simulink model "SwarmSystem_2021b"  (R2021b)
settings: Solver=VariableStepAuto  StartTime=0.0  StopTime=10.0  RelTol=1e-3
values from neighbouring files (symbols this model uses):
  dt = 0.01    [init_params.m]
  initial_state_x0 = Simulink.Parameter(initial_state_x0)    [init_params.m]    (also in single_model_verification_script.m = [W0; R0; dP0; P0]; team_model_conf_comp_script.m = [W0; R0; dP0; P0]; team_model_tethered_tilt.m = [W0; R0; dP0; P0]; team_model_tracking_script.m = [W0; R0; dP0; P0])
undefined symbols (not defined in the file or in its folder): ctrl_params, drone_params, env_params, initial_state_z0
libraries: dspindex x15
settings Model: Creator=NTU  LastModifiedBy=NTU
settings DataIOCC: SaveFinalState=on  SaveState=on
settings DebuggingCC: UnconnectedInputMsg=none  UnconnectedOutputMsg=none  UnconnectedLineMsg=none
settings ModelReferenceCC: EnableRefExpFcnMdlSchedulingChecks=off
settings RTWCC: DLArmComputeVersion=20.02.1

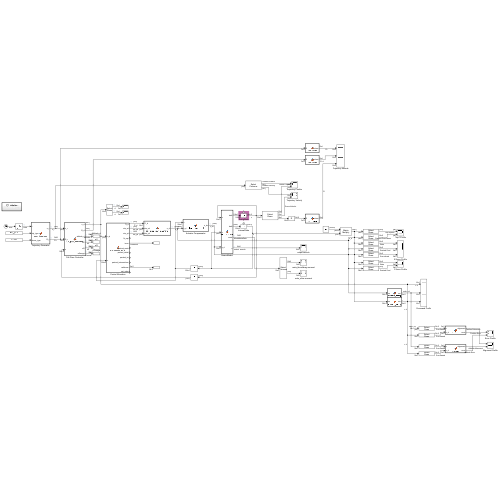
[thumbnail: Simulink's stored preview of the top-level diagram]
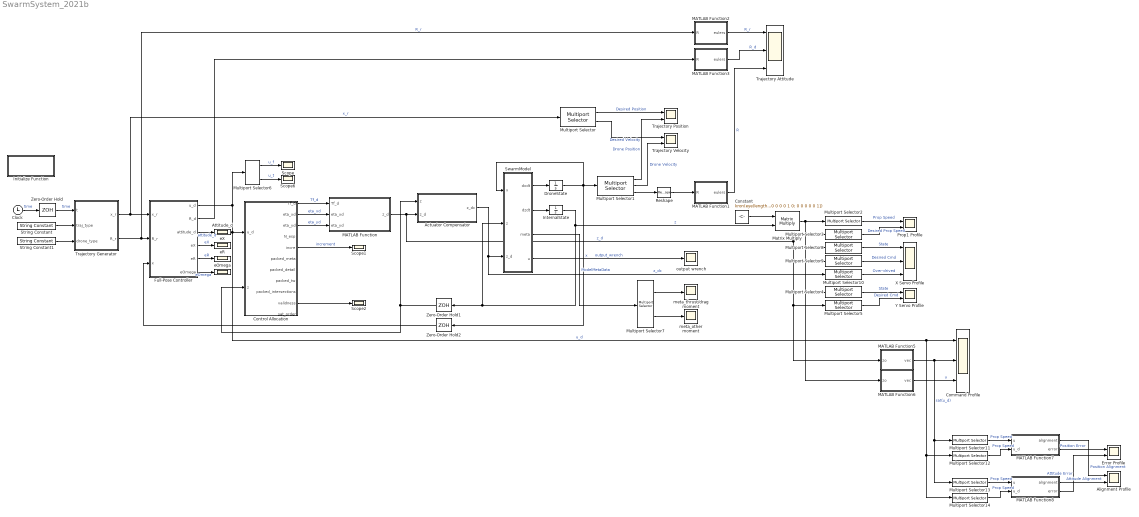
== system SwarmSystem_2021b ==
  Actuator Compensator : MATLAB Function  TreatAsAtomicUnit=on
  Alignment Profile : Scope  NumInputPorts=2
  Attitude_d : Scope
  Clock : Clock
  Command Profile : Scope  NumInputPorts=3
  Constant : Constant  Value=kron(eye(length(drone_params.psi)), [1 0 0 0 0 0;0 0 1 0 0 0; 0 0 0 0 1 0; 0 0 0 0 0 1])  VectorParams1D=off
  Control Allocation : MATLAB Function  TreatAsAtomicUnit=on
  DroneState : Integrator  InitialCondition=zeros([18 1])  ContinuousStateAttributes='x'
  Error Profile : Scope  NumInputPorts=2
  Full-Pose Controller : MATLAB Function  TreatAsAtomicUnit=on
  Initialize Function : Subsystem  TreatAsAtomicUnit=on
  InternalState : Integrator  InitialCondition=zeros([6*length(drone_params.psi) 1])  ContinuousStateAttributes='z'
  MATLAB Function : MATLAB Function  TreatAsAtomicUnit=on
  MATLAB Function1 : MATLAB Function  TreatAsAtomicUnit=on
  MATLAB Function2 : MATLAB Function  TreatAsAtomicUnit=on
  MATLAB Function3 : MATLAB Function  TreatAsAtomicUnit=on
  MATLAB Function5 : MATLAB Function  TreatAsAtomicUnit=on
  MATLAB Function6 : MATLAB Function  TreatAsAtomicUnit=on
  MATLAB Function7 : MATLAB Function  TreatAsAtomicUnit=on
  MATLAB Function8 : MATLAB Function  TreatAsAtomicUnit=on
  Matrix Multiply : Product  Multiplication=Matrix(*)
  Multiport Selector : dspindex/Multiport Selector  rowsOrCols=Columns  idxCellArray={ 1, 2 }  idxErrMode=Clip Index
  Multiport Selector1 : dspindex/Multiport Selector  rowsOrCols=Rows  idxCellArray={ [16:18], [13:15], [4:12] }  idxErrMode=Clip Index
  Multiport Selector10 : dspindex/Multiport Selector  rowsOrCols=Rows  idxCellArray={ [4 8 12 16 20 24 28 32 36]-3 }  idxErrMode=Clip Index
  Multiport Selector11 : dspindex/Multiport Selector  rowsOrCols=Rows  idxCellArray={ [1:3]}  idxErrMode=Clip Index
  Multiport Selector12 : dspindex/Multiport Selector  rowsOrCols=Rows  idxCellArray={ [1:3]}  idxErrMode=Clip Index
  Multiport Selector13 : dspindex/Multiport Selector  rowsOrCols=Rows  idxCellArray={ [4:6]}  idxErrMode=Clip Index
  Multiport Selector14 : dspindex/Multiport Selector  rowsOrCols=Rows  idxCellArray={ [4:6]}  idxErrMode=Clip Index
  Multiport Selector2 : dspindex/Multiport Selector  rowsOrCols=Rows  idxCellArray={ [4 8 12 16 20 24 28 32 36]-1 }  idxErrMode=Clip Index
  Multiport Selector3 : dspindex/Multiport Selector  rowsOrCols=Rows  idxCellArray={ [4 8 12 16 20 24 28 32 36]-1 }  idxErrMode=Clip Index
  Multiport Selector4 : dspindex/Multiport Selector  rowsOrCols=Rows  idxCellArray={ [4 8 12 16 20 24 28 32 36]-2 }  idxErrMode=Clip Index
  Multiport Selector5 : dspindex/Multiport Selector  rowsOrCols=Rows  idxCellArray={ [4 8 12 16 20 24 28 32 36]-2 }  idxErrMode=Clip Index
  Multiport Selector6 : dspindex/Multiport Selector  rowsOrCols=Rows  idxCellArray={ [1:3], [4:6] }  idxErrMode=Clip Index
  Multiport Selector7 : dspindex/Multiport Selector  rowsOrCols=Columns  idxCellArray={ [1:2], [3:5]}  idxErrMode=Clip Index
  Multiport Selector8 : dspindex/Multiport Selector  rowsOrCols=Rows  idxCellArray={ [4 8 12 16 20 24 28 32 36]-3 }  idxErrMode=Clip Index
  Multiport Selector9 : dspindex/Multiport Selector  rowsOrCols=Rows  idxCellArray={ [4 8 12 16 20 24 28 32 36]-3 }  idxErrMode=Clip Index
  Prop1 Profile : Scope  NumInputPorts=2
  Reshape : Reshape  OutputDimensionality=Customize  OutputDimensions=[3,3]
  Scope{,1..2,6} (4 alike) : Scope
  String Constant : StringConstant  String=traj_type
  String Constant1 : StringConstant  String="\"team\""
  SwarmModel : MATLAB Function  TreatAsAtomicUnit=on
  Trajectory Attitude : Scope  NumInputPorts=3
  Trajectory Generator : MATLAB Function  TreatAsAtomicUnit=on
  Trajectory Position : Scope  NumInputPorts=2
  Trajectory Velocity : Scope  NumInputPorts=2
  X Servo Profile : Scope  NumInputPorts=3
  Y Servo Profile : Scope  NumInputPorts=2
  Zero-Order Hold : ZeroOrderHold  SampleTime=dt
  Zero-Order Hold1 : ZeroOrderHold  SampleTime=dt
  Zero-Order Hold2 : ZeroOrderHold  SampleTime=dt
  eOmega : Scope
  eR : Scope
  eX : Scope
  meta_other moment : Scope
  meta_thrust/drag moment : Scope
  output wrench : Scope
  wires:
  SwarmModel/1(dxdt) -> DroneState/1
  Clock/1 -> Zero-Order Hold/1  "time"
  Trajectory Generator/1(x_r) -> Multiport Selector/1, Full-Pose Controller/1(x_r)  "x_r"
  Trajectory Generator/2(R_r) -> MATLAB Function2/1(R), Full-Pose Controller/2(R_r)  "R_r"
  Multiport Selector/1 -> Trajectory Position/1  "Desired Position"
  Multiport Selector1/1 -> Trajectory Position/2  "Drone Position"
  Multiport Selector1/2 -> Trajectory Velocity/2  "Drone Velocity"
  Multiport Selector/2 -> Trajectory Velocity/1  "Desired Velocity"
  Multiport Selector2/1 -> Prop1 Profile/1  "Prop Speed"
  SwarmModel/2(dzdt) -> InternalState/1
  Control Allocation/1(Tf_d) -> MATLAB Function/1(Tf_d)  "Tf_d"
  Control Allocation/2(eta_xd) -> MATLAB Function/2(eta_xd)  "eta_xd"
  Control Allocation/3(eta_yd) -> MATLAB Function/3(eta_yd)  "eta_yd"
  MATLAB Function/1(z_d) -> Multiport Selector3/1, MATLAB Function5/1(zo), Multiport Selector5/1, Multiport Selector9/1, Actuator Compensator/2(z_d)  "z_d"
  DroneState/1 -> SwarmModel/1(x), Zero-Order Hold2/1, Multiport Selector1/1  "x"
  InternalState/1 -> Zero-Order Hold1/1, SwarmModel/2(z), Matrix Multiply/2  "z"
  Multiport Selector6/1 -> Scope/1  "u_f"
  Multiport Selector6/2 -> Scope6/1  "u_t"
  MATLAB Function1/1(eulers) -> Trajectory Attitude/3  "R"
  Multiport Selector1/3 -> Reshape/1
  Reshape/1 -> MATLAB Function1/1(R)
  MATLAB Function2/1(eulers) -> Trajectory Attitude/1  "R_r"
  Full-Pose Controller/2(R_d) -> MATLAB Function3/1(R)
  MATLAB Function3/1(eulers) -> Trajectory Attitude/2  "R_d"
  Constant/1 -> Matrix Multiply/1
  MATLAB Function6/1(vec) -> Command Profile/3  "u"
  Multiport Selector3/1 -> Prop1 Profile/2  "Desired Prop Speed"
  Multiport Selector8/1 -> X Servo Profile/1  "State"
  Multiport Selector9/1 -> X Servo Profile/2  "Desired Cmd"
  Multiport Selector5/1 -> Y Servo Profile/2  "Desired Cmd"
  Multiport Selector4/1 -> Y Servo Profile/1  "State"
  Matrix Multiply/1 -> MATLAB Function6/1(zo), Multiport Selector4/1, Multiport Selector8/1, Multiport Selector2/1
  Zero-Order Hold/1 -> Trajectory Generator/1(t)  "time"
  Actuator Compensator/1(z_dc) -> Multiport Selector10/1, SwarmModel/3(z_d)  "z_dc"
  Multiport Selector10/1 -> X Servo Profile/3  "Over-drived"
  Zero-Order Hold1/1 -> Actuator Compensator/1(z), Control Allocation/2(z)
  Zero-Order Hold2/1 -> Full-Pose Controller/3(x)
  Multiport Selector11/1 -> MATLAB Function7/1(u)  "Prop Speed"
  Multiport Selector12/1 -> MATLAB Function7/2(u_d)  "Prop Speed"
  Multiport Selector14/1 -> MATLAB Function8/2(u_d)  "Prop Speed"
  Multiport Selector13/1 -> MATLAB Function8/1(u)  "Prop Speed"
  Full-Pose Controller/1(u_d) -> Multiport Selector12/1, Multiport Selector14/1, Command Profile/1, Control Allocation/1(u_d), Multiport Selector6/1  "u_d"
  MATLAB Function5/1(vec) -> Multiport Selector13/1, Multiport Selector11/1, Command Profile/2  "sat(u_d)"
  MATLAB Function7/2(error) -> Error Profile/1  "Position Error"
  MATLAB Function8/2(error) -> Error Profile/2  "Attitude Error"
  MATLAB Function7/1(alignment) -> Alignment Profile/1  "Position Alignment"
  MATLAB Function8/1(alignment) -> Alignment Profile/2  "Attitude Alignment"
  Control Allocation/5(incre) -> Scope1/1  "increment"
  Control Allocation/10(validness) -> Scope2/1
  String Constant/1 -> Trajectory Generator/2(traj_type)
  String Constant1/1 -> Trajectory Generator/3(drone_type)
  Full-Pose Controller/4(eX) -> eX/1  "eX"
  Full-Pose Controller/6(eOmega) -> eOmega/1  "eOmega"
  Full-Pose Controller/5(eR) -> eR/1  "eR"
  Full-Pose Controller/3(attitude_d) -> Attitude_d/1  "attitude_d"
  Multiport Selector7/2 -> meta_other moment/1
  Multiport Selector7/1 -> meta_thrust/drag moment/1
  SwarmModel/3(meta) -> Multiport Selector7/1  "ModelMetaData"
  SwarmModel/4(u) -> output wrench/1  "output_wrench"

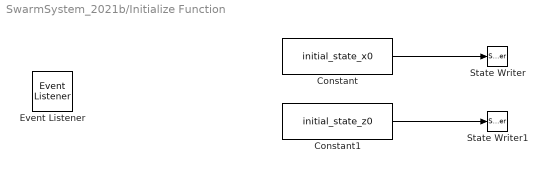
== system SwarmSystem_2021b/Initialize Function ==
  Constant : Constant  Value=initial_state_x0  VectorParams1D=off
  Constant1 : Constant  Value=initial_state_z0  VectorParams1D=off
  Event Listener : EventListener  DisableCoverage=on  EventName=reset
  State Writer : StateWriter  StateOwnerBlock=../../DroneState  StateName=x
  State Writer1 : StateWriter  StateOwnerBlock=../../InternalState  StateName=z
  wires:
  Constant/1 -> State Writer/1
  Constant1/1 -> State Writer1/1

== matlab function SwarmSystem_2021b/MATLAB Function2 ==
  data: R input; eulers output
function eulers = rotm2euler(R)
    psi = atan2(-R(1, 2), R(2, 2));    
    phi = atan2(R(3, 2), sqrt(abs(1-R(3, 2).^2)));
    theta = atan2(-R(3, 1), R(3, 3));
    eulers = [psi phi theta]';
end

== matlab function SwarmSystem_2021b/MATLAB Function3 ==
  data: R input; eulers output
function eulers = rotm2euler(R)
    psi = atan2(-R(1, 2), R(2, 2));    
    phi = atan2(R(3, 2), sqrt(abs(1-R(3, 2).^2)));
    theta = atan2(-R(3, 1), R(3, 3));
    eulers = [psi phi theta]';
end

== matlab function SwarmSystem_2021b/MATLAB Function5 ==
  data: zo input; drone_params parameter; vec output; env_params parameter
function vec = actuator_mixing(zo, drone_params, env_params)
    %% Parameters
    g = env_params.g; % gravity
    rho = env_params.rho; % kg/m3
    prop_d = env_params.prop_d; % 8 inch = 20.3 cm
    
    CT_u = env_params.CT_u; % upper propeller thrust coefficient
    CT_l = env_params.CT_l; % lower propeller thrust coefficient
    CP_u = env_params.CP_u; % upper propeller drag coefficient
    CP_l = env_params.CP_l; % lower propeller drag coefficient

    pos = drone_params.pos;
    psi = drone_params.psi;
    n = length(psi);

    Tf = zeros([n 1]);
    eta_x = zeros([n 1]);
    eta_y = zeros([n 1]);

    beta_allo = [CT_u CT_l; prop_d * CP_u -prop_d * CP_l];
    P_prop = rho * prop_d^4 * beta_allo;

    for i = 1:n
        % Actuator Model
        zi = zo(4 * (i - 1) + 1 : 4 * i);
        TfTdi = P_prop * zi(3:4, 1).^2;
        Tf(i) = TfTdi(1);
        eta_x(i) = zi(1);
        eta_y(i) = zi(2);
    end

    M = get_M(n, psi, pos);
    fi = get_f(eta_x, eta_y, Tf);
    vec = M * fi;
end

== matlab function SwarmSystem_2021b/MATLAB Function6 ==
  data: zo input; drone_params parameter; vec output; env_params parameter
function vec = actuator_mixing(zo, drone_params, env_params)
    %% Parameters
    g = env_params.g; % gravity
    rho = env_params.rho; % kg/m3
    prop_d = env_params.prop_d; % 8 inch = 20.3 cm
    
    CT_u = env_params.CT_u; % upper propeller thrust coefficient
    CT_l = env_params.CT_l; % lower propeller thrust coefficient
    CP_u = env_params.CP_u; % upper propeller drag coefficient
    CP_l = env_params.CP_l; % lower propeller drag coefficient

    pos = drone_params.pos;
    psi = drone_params.psi;
    n = length(psi);

    Tf = zeros([n 1]);
    eta_x = zeros([n 1]);
    eta_y = zeros([n 1]);

    beta_allo = [CT_u CT_l; prop_d * CP_u -prop_d * CP_l];
    P_prop = rho * prop_d^4 * beta_allo;

    for i = 1:n
        % Actuator Model
        zi = zo(4 * (i - 1) + 1 : 4 * i);
        TfTdi = P_prop * zi(3:4, 1).^2;
        Tf(i) = TfTdi(1);
        eta_x(i) = zi(1);
        eta_y(i) = zi(2);
    end

    M = get_M(n, psi, pos);
    fi = get_f(eta_x, eta_y, Tf);
    vec = M * fi;
end

== matlab function SwarmSystem_2021b/Actuator Compensator ==
  settings: updateMethod=DISCRETE  sampleTime=dt
  data: z input; z_d input; z_dc output; drone_params parameter; dt parameter
function z_dc = acutator_compensator(z, z_d, drone_params, dt)
    psi = drone_params.psi;
    n = length(psi);    
    
    mKp = drone_params.mKp; % Servo motor gain
    mKd = drone_params.mKd; % Servo motor gain
    pKp = drone_params.pKp; % BLDC motor gain

    sigma_x = drone_params.sigma_a;
    sigma_y = drone_params.sigma_b;
    z_dc = opt_compensator(n, z, z_d, sigma_x, sigma_y);
    %z_dc = compensator(n, z, z_d, dt, mKp, mKd, sigma_x, sigma_y);
end

function z_dc = opt_compensator(n, z, z_d, sigma_x, sigma_y)
    z_dc = z_d;
    for i=1:n
        zi = z(6*(i-1)+1 : 6*i);
        x_zi = [1 0 0 0 0 0; 0 0 1 0 0 0] * zi;
        v_zi = [0 1 0 0 0 0; 0 0 0 1 0 0] * zi;

        z_di = z_d(4*(i-1)+1 : 4*(i-1)+2);
        %z_dcr = -14.3636 * (x_zi-z_di) - 0.3070 * (v_zi-0) + 0.6924 * z_di;
        z_dcr = -28.0209 * (x_zi-z_di) -0.5379 * (v_zi-0) + 0.9971 * z_di;
        %z_dcr = -17.3915 * (x_zi-z_di) -0.4492 * (v_zi-0) + 0.8054 * z_di;
        %z_dcr = -11.8288 * (x_zi-z_di) -0.4958 * (v_zi-0) + 0.4905 * z_di;
        
        z_dcr(1) = min(sigma_x, max(-sigma_x, z_dcr(1)));
        z_dcr(2) = min(sigma_y, max(-sigma_y, z_dcr(2)));

        z_dc(4*(i-1)+1 : 4*(i-1)+2) = z_dcr;
    end
end

function z_dc = compensator(n, z, z_d, dt, mKp, mKd, sigma_x, sigma_y)
    w_n = sqrt(mKp);
    zeta = mKd / (2 * w_n);
    k = mKp;

    w_d = w_n * sqrt(1 - zeta^2);
    sigma = -zeta * w_n;

    C1 = (w_n / w_d) * exp(sigma * dt) * sin(w_d * dt + atan(w_d / -sigma));
    C2 = (exp(sigma * dt) / w_d) * sin(w_d * dt);
    C3 = (k / w_d) * (w_d + exp(sigma * dt) * (sigma*sin(w_d*dt) - w_d*cos(w_d*dt))) / w_n^2;

    z_dc = z_d;
    %return
    
    for i=1:n
        zi = z(6*(i-1)+1 : 6*i);
        x_zi = [1 0 0 0 0 0; 0 0 1 0 0 0] * zi;
        v_zi = [0 1 0 0 0 0; 0 0 0 1 0 0] * zi;

        z_di = z_d(4*(i-1)+1 : 4*(i-1)+2);
        delta_z_di = z_di - x_zi;

        M = (delta_z_di + (1-C3-C1)*x_zi - C2*v_zi) ./ (C3 * delta_z_di);
        z_dcr = x_zi + delta_z_di .* M;
        
        z_dcr(1) = min(sigma_x, max(-sigma_x, z_dcr(1)));
        z_dcr(2) = min(sigma_y, max(-sigma_y, z_dcr(2)));

        z_dc(4*(i-1)+1 : 4*(i-1)+2) = z_dcr;
    end
end

== matlab function SwarmSystem_2021b/MATLAB Function7 ==
  data: u input; alignment output; u_d input; error output
function [alignment, error] = metrices(u, u_d)
    error = norm(u_d - u) / norm(u_d);
    alignment = u' * u_d / (norm(u_d) * norm(u));
end

== matlab function SwarmSystem_2021b/MATLAB Function8 ==
  data: u input; alignment output; u_d input; error output
function [alignment, error] = metrices(u, u_d)
    error = norm(u_d - u) / norm(u_d);
    alignment = u' * u_d / (norm(u_d) * norm(u));
end

== matlab function SwarmSystem_2021b/Full-Pose Controller ==
  settings: updateMethod=DISCRETE  sampleTime=dt
  data: x_r input; u_d output size=[6 1]; R_r input; x input; env_params parameter; drone_params parameter; R_d output; attitude_d output; eX output; eR output; eOmega output; ctrl_params parameter
function [u_d, R_d, attitude_d, eX, eR, eOmega] = full_pose_controller(x_r, R_r, x, env_params, drone_params, ctrl_params)
    m = drone_params.mb; % Mass, Kg
    g = env_params.g;
    I_b = drone_params.I_b; % Leverage length from c.p. to c.g.
    
    % States
    p = x(16:18);
    v = x(13:15);
    R = reshape(x(4:12), [3 3]); % 3x3
    w = x(1:3);
    
    % Gain
    Kp = ctrl_params.Kp;
    Kd = ctrl_params.Kd;
    Kr = ctrl_params.Kr;
    Ko = ctrl_params.Ko;
    
    % % Translational error
    ep = p - x_r(1:3, 1);
    ev = v - x_r(1:3, 2);
    eX = [ep ev];
    
    f_r = m * x_r(1:3, 3) + m*[0; 0; g] + m * (- Kp * ep - Kd * ev);
    u_f = R' * f_r;
    u_f = force_sat(drone_params, u_f);
    
    [R_d, theta] = calc_R_d(drone_params, f_r, R_r);
    %R_d = R_r;
    % w_d = vee(R_d' * d_R_d);
    
    % Attitude error
    eRx = 0.5 * (R_d' * R - R' * R_d);
    eR = vee(eRx);
    % eOmega = w - R' * R_d * w_d;
    eOmega = w;
    attitude_d = rot2zxy(R_d);
    
    u_tau = cross(w, I_b * w) + I_b * ( - Kr * eR - Ko * eOmega);
    u_d = [u_f; u_tau];
end

function u_sat = force_sat(drone_params, u)
    psi = drone_params.psi;
    sigma_a = drone_params.sigma_a;
    f_max = drone_params.f_max;
    n = length(psi);

    n_x = sum(psi == 0);
    n_y = n - n_x;

    a = n_x * f_max + (n_y ~= 0) * u(3) * tan(sigma_a);
    b = n_y * f_max + (n_x ~= 0) * u(3) * tan(sigma_a);
    t = (a * b) / sqrt(u(1)^2 * b^2 + u(2)^2 * a^2);

    % Directional saturation
    u_sat = u;
    if t < 1
        u_sat(1:2) = t * u(1:2);
    end

    % Magnitude saturation
    roof_lim = n * drone_params.f_max;
    scale = norm(u_sat(1:3)) / roof_lim;
    if scale > 1
        u_sat(1:3) = u_sat(1:3) / scale;
    end
end

function [R_d, theta] = calc_R_d(drone_params, f_r, R_r)
    b1r = R_r(:, 1);
    b2r = R_r(:, 2);
    b3r = R_r(:, 3);
    [theta] = ctrl_sat_square_bisection(drone_params, 20, b1r, b3r, f_r);

    k = cross(b3r, f_r) / norm(cross(b3r, f_r));
    nb3 = rot_vec_by_theta(b3r, k, theta);
    nb2 = cross(nb3, b1r) / norm(cross(nb3, b1r));
    nb1 = cross(nb2, nb3);
    R_d = [nb1 nb2 nb3];
end

function [theta] = ctrl_sat_square_bisection(drone_params, n, b1r, b3r, f_r)
    %sigma_a = conf('sigma_a');
    b2r = cross(b3r, b1r);
    theta_max = acos(b3r' * f_r / norm(f_r));
    % theta_max = asin(norm(cross(b3r, f_r)) / norm(f_r));
    theta = theta_max / 2;
    % abs(f_r' * b2r)
    % f_r' * b3r * tan(sigma_a)
    % if abs(f_r' * b2r) > f_r' * b3r * tan(sigma_a)
    if ~is_attainable(drone_params, b1r, b2r, b3r, f_r)
        k = cross(b3r, f_r) / norm(cross(b3r, f_r));
        for i=1:n
            b3 = rot_vec_by_theta(b3r, k, theta);
            b2 = cross(b3, b1r) / norm(cross(b3, b1r));
            b1 = cross(b2, b3);
            % if abs(f_r' * b2) < f_r' * b3 * tan(sigma_a)
            if is_attainable(drone_params, b1, b2, b3, f_r)
                theta = theta - 0.5 * theta_max / (2^i);
            else
                theta = theta + 0.5 * theta_max / (2^i);
            end
            % fprintf("%d: %.4f\n", i, theta)
        end
    else
        theta = 0;
    end
end

function out = rot_vec_by_theta(vec, rot_axis, theta)
    out = vec * cos(theta) + cross(rot_axis, vec) * sin(theta) + rot_axis * (rot_axis' * vec) * (1 - cos(theta));
end

function feasible = is_attainable(drone_params, b1, b2, b3, f_r)
    feasible = elliptic_cone(drone_params, b1, b2, b3, f_r);
    % feasible = pie(conf, b1, b2, b3, f_r);
end

function feasible = elliptic_cone(drone_params, b1, b2, b3, f_r)
    n = length(drone_params.psi);
    f_max = drone_params.f_max;
    sigma_a = drone_params.sigma_a;
    sigma_b = drone_params.sigma_b;

    n_x = sum(drone_params.psi == 0);
    n_y = n - n_x;

    z = f_r' * b3;
    c_x = fun_g(n_x, sigma_b, z, f_max) + fun_g(n_y, sigma_a, z, f_max);
    c_y = fun_g(n_x, sigma_a, z, f_max) + fun_g(n_y, sigma_b, z, f_max);

    feasible = (z > 0) & (((f_r' * b1 / c_x)^2 + (f_r' * b2 / c_y)^2) <= 1);
end

function gk = fun_g(n_k, sigma_k_bar, z, f_max)
    if (sigma_k_bar >= pi / 2)
        gk = n_k * f_max;
    else
        gk = (n_k > 0) * z * tan(sigma_k_bar);
    end
end

== matlab function SwarmSystem_2021b/SwarmModel ==
  data: x input; z input; dxdt output; z_d input; dzdt output; env_params parameter; drone_params parameter; meta output; u output
function [dxdt, dzdt, meta, u] = swarm_model(x, z, z_d, env_params, drone_params)
   %[dxdt, dzdt, meta, u] = tvmd_model(x, z, z_d, env_params, drone_params);
   [dxdt, dzdt, meta, u] = tvmd_model_RNEA(x, z, z_d, env_params, drone_params);
end

== matlab function SwarmSystem_2021b/Control Allocation ==
  settings: updateMethod=DISCRETE  sampleTime=dt
  data: Tf_d output size=[9 1]; u_d input; eta_xd output; eta_yd output; z input; drone_params parameter; env_params parameter; dt parameter; N_esp output; incre output; packed_meta output; packed_detail output; packed_tw output; packed_intersections output; validness output; sat_order output
function [Tf_d, eta_xd, eta_yd, N_esp, incre, packed_meta, packed_detail, packed_tw, packed_intersections, validness, sat_order] = ControlAllocation(u_d, z, drone_params, env_params, dt)
    sigma_x = drone_params.sigma_a;
    sigma_y = drone_params.sigma_b;
    f_max = drone_params.f_max;

    %[Tf_d, eta_xd, eta_yd] = allocator_moore_penrose(env_params, drone_params, u_d, z, dt);
    %N_esp = 0; incre = 0; packed_meta = 0; validness = 0;
    %packed_meta=0; packed_detail=0; packed_tw=0; packed_intersections=0; sat_order=0;
    [Tf_d, eta_xd, eta_yd, N_esp, incre, packed_meta, packed_detail, packed_tw, packed_intersections, validness, sat_order] = allocator_redistributed_nonlinear(env_params, drone_params, u_d, z, dt);
    %[Tf_d, eta_xd, eta_yd] = allocator_interior_point(drone_params, u_d, z);

    Tf_d = min(f_max, max(0, Tf_d));
    eta_xd = min(sigma_x, max(-sigma_x, eta_xd));
    eta_yd = min(sigma_y, max(-sigma_y, eta_yd));
end

== matlab function SwarmSystem_2021b/MATLAB Function ==
  settings: updateMethod=DISCRETE  sampleTime=dt
  data: Tf_d input; z_d output; eta_xd input; eta_yd input; env_params parameter; drone_params parameter
function z_d = calc_prop_raw_command(Tf_d, eta_xd, eta_yd, env_params, drone_params)
    % Parameters
    rho = env_params.rho; % kg/m3
    prop_d = env_params.prop_d; % 8 inch = 20.3 cm

    CT_u = env_params.CT_u; % upper propeller thrust coefficient
    CT_l = env_params.CT_l; % lower propeller thrust coefficient
    CP_u = env_params.CP_u; % upper propeller drag coefficient
    CP_l = env_params.CP_l; % lower propeller drag coefficient

    sigma_x = drone_params.sigma_a;
    sigma_y = drone_params.sigma_b;
    sigma_w0 = drone_params.sigma_w0;
    sigma_w = drone_params.prop_max;

    psi = drone_params.psi;
    n = length(psi);

    % Inversing
    beta_allo = [CT_u CT_l; prop_d * CP_u -prop_d * CP_l];

    z_d = zeros([4*n 1]);
    for i=1:n
        wm_d = sqrt(beta_allo \ [Tf_d(i); 0] / (rho * prop_d^4));
        z_di = [eta_xd(i); eta_yd(i); wm_d];

        z_low = [-sigma_x; -sigma_y;   sigma_w0;    sigma_w0];
        z_upp = [ sigma_x;  sigma_y; sigma_w(1);  sigma_w(2)];
        z_d(4*(i-1)+1 : 4*i) = min(z_upp, max(z_low, z_di));
    end
end

== matlab function SwarmSystem_2021b/Trajectory Generator ==
  data: t input; x_r output; R_r output; traj_type input; drone_type input; traj_params parameter
function [x_r, R_r] = gen_trajectory(t, traj_type, drone_type, traj_params)
    coder.extrinsic('init_traj');
    traj_func = zeros([6 3]);
    traj_func = init_traj(t, traj_type, drone_type, traj_params);
    traj = traj_func;
    x_r = traj(1:3, :);

    psi_d = traj(4, 1); phi_d = traj(5, 1); theta_d = traj(6, 1);
    R_r = getI_R_B(psi_d, phi_d, theta_d);
end

== matlab function SwarmSystem_2021b/MATLAB Function1 ==
  data: R input; eulers output
function eulers = rotm2euler(R)
    psi = atan2(-R(1, 2), R(2, 2));    
    phi = atan2(R(3, 2), sqrt(abs(1-R(3, 2).^2)));
    theta = atan2(-R(3, 1), R(3, 3));
    eulers = [psi phi theta]';
end
